simulink model "GS_model"  (R2018b)
settings: Solver=ode5  StartTime=0.0  StopTime=SimuStopTime  FixedStep=T_Simu  RelTol=1e-3
InitFcn:
  | Initial
undefined symbols (not defined in the file or in its folder): Aba10, Aba20, aeroCIP2006_S, aeroCIP2006_X, aeroCIP2006_Y, Agl0, Ass_kS, Ass_n1, Ass_n2, Ass_n3, Ass_n4, Ass_Noise, Ass_R, Ass_Resolution, Ass_TmOrder, AssA_Fix_Abs, AssB_Fix_Abs, AssC_Fix_Abs, AssD_Fix_Abs, AssE_Fix_Aps, AssF_Fix_Aps, C, c_max, c_min, Cd, CenterOfFigNX, CenterOfFigNY, CenterOfFigNZ, CenterOfFigP1, CenterOfFigP2, CenterOfFigPX, CenterOfFigPY, CenterOfFigPZ, Cmu, Crou, DEG2RAD, DiscIntNeverNeededParam, Eg_Dir, Eg_F, Eg_PrepareTime, Eg_r_L_L, Fw_Abf, Fw_Hmax, Fw_J, Fw_Spd0, Fw_Tmax, git_hash_BaseLine, git_hash_Project, Gnss_Noise_Pos, Gnss_Noise_Vel, Gnss_PropgationTime, GyroA_Fix_Abg, GyroA_Noise, GyroB_Fix_Abg, GyroB_Noise, GyroC_Fix_Abg, GyroC_Noise, GyroD_Fix_Abg, GyroD_Noise, h ... (+94)
libraries: simulink x308, sharedutil x46, aerolibutil x37, sharedtransform x31, vrlib x14, aerolibgravity2 x2
(part 19 of 20)

== matlab function GS_model/Subsystem2/Subsystem/Actuator/Motor/SADA/MATLAB Function4 ==
  settings: updateMethod=DISCRETE
  data: Tc_level output; u input; InitialAgl output
function [Tc_level , InitialAgl] =Initial(u)
Tc_AglSetEnable = u(1);
Tc_AglSetValue = u(2:7);
Tc_Reset = u(8);
Tc_Reset_Agl = u(9:14);
DataSource = u(15:20);
Agl_FC = u(21:26);
%% 输入变量、局部变量定义
persistent Tc_AglSetEnable_last DATA_Motor_Agl;

if isempty(Tc_AglSetEnable_last) || Tc_Reset == 1    %3322
    Tc_AglSetEnable_last = 0;
end
if isempty(DATA_Motor_Agl) || Tc_Reset == 1    %3322
    DATA_Motor_Agl = [0;0;0;0;0;0];
end
%% 动力学初始角度设置
if Tc_AglSetEnable_last == 0 && Tc_AglSetEnable == 1  %动力学遥控 
    Tc = [1;1;1;1;1;1];
    DATA_Motor_Agl = Tc_AglSetValue;
elseif Tc_Reset == 1 
    Tc = [1;1;1;1;1;1];
    DATA_Motor_Agl = Tc_Reset_Agl;
else
    Tc = double(DataSource==[1;1;1;1;1;1]);
    for i = 1:6
        if Tc(i) == 1 % 真采集时，取反测值
            DATA_Motor_Agl(i)  = Agl_FC(i);
        end
    end
end

Tc_AglSetEnable_last = Tc_AglSetEnable;
InitialAgl= DATA_Motor_Agl;
Tc_level =Tc;
end

== matlab function GS_model/Subsystem2/Subsystem/Actuator/Motor/QV/MATLAB Function4 ==
  settings: updateMethod=DISCRETE
  data: Tc_level output; u input; InitialAgl output
function [Tc_level , InitialAgl] =Initial(u)
Tc_AglSetEnable = u(1);
Tc_AglSetValue = u(2:5);
Tc_Reset = u(6);
Tc_Reset_Agl = u(7:10);
DataSource = u(11:14);
Agl_FC = u(15:18);
%% 输入变量、局部变量定义
persistent Tc_AglSetEnable_last DATA_Motor_Agl;

if isempty(Tc_AglSetEnable_last) || Tc_Reset == 1    %3322
    Tc_AglSetEnable_last = 0;
end
if isempty(DATA_Motor_Agl) || Tc_Reset == 1    %3322
    DATA_Motor_Agl = [0;0;0;0];
end
%% 动力学初始角度设置
if Tc_AglSetEnable_last == 0 && Tc_AglSetEnable == 1  %动力学遥控 
    Tc = [1;1;1;1];
    DATA_Motor_Agl = Tc_AglSetValue;
elseif Tc_Reset == 1 
    Tc = [1;1;1;1];
    DATA_Motor_Agl = Tc_Reset_Agl;
else
    Tc = double(DataSource==[1;1;1;1]);
    for i = 1:4
        if Tc(i) == 1 % 真采集时，取反测值
            DATA_Motor_Agl(i)  = Agl_FC(i);
        end
    end
end

Tc_AglSetEnable_last = Tc_AglSetEnable;
InitialAgl= DATA_Motor_Agl;
Tc_level =Tc;
end

== matlab function GS_model/Subsystem2/Subsystem/Sensor/GNSS/Orbit/MATLAB Function2 ==
  data: RV_i output; Orbit input
function RV_i = Orbit2RV(Orbit)
% 瞬根轨道转惯性系RV
a = Orbit(1);
e = Orbit(2);
i = Orbit(3);
OMG = Orbit(4);
omg = Orbit(5);
f = Orbit(6);
p=a*(1-e^2);
r0=p/(1+e*cos(f));
miu = 3.9860044e14;
% v0=sqrt(mu*(2/r0-1/a));
% sg=e*sin(f)/sqrt(1+e^2+2*e*cos(f));
% cg=sqrt(1-sg^2);
x0=r0*(cos(omg+f)*cos(OMG)-sin(omg+f)*cos(i)*sin(OMG));
y0=r0*(cos(omg+f)*sin(OMG)+sin(omg+f)*cos(i)*cos(OMG));
z0=r0*sin(omg+f)*sin(i);
R_i = [x0;y0;z0];
% x0=1184844.6264962;y0=-3166067.5090052;z0=6192267.2136932;
% vx0=v0*(sg*(cos(omg+f)*cos(OMG)-sin(omg+f)*cos(i)*sin(OMG))+cg*(-sin(omg+f)*cos(OMG)-cos(omg+f)*cos(i)*sin(OMG)));% x肖业伦P53
% vy0=v0*(sg*(cos(omg+f)*sin(OMG)+sin(omg+f)*cos(i)*cos(OMG))+cg*(-sin(omg+f)*sin(OMG)+cos(omg+f)*cos(i)*cos(OMG)));
% vz0=v0*(sg*sin(omg+f)*sin(i)+cg*cos(omg+f)*sin(i));
sp=[cos(omg)*cos(OMG)-sin(omg)*sin(OMG)*cos(i);cos(omg)*sin(OMG)+sin(omg)*cos(OMG)*cos(i);sin(omg)*sin(i)];
sq=[-sin(omg)*cos(OMG)-cos(omg)*sin(OMG)*cos(i);-sin(omg)*sin(OMG)+cos(omg)*cos(OMG)*cos(i);cos(omg)*sin(i)];
vx0=sqrt(miu/a/(1-e^2))*(-sin(f)*sp(1)+(e+cos(f))*sq(1));
vy0=sqrt(miu/a/(1-e^2))*(-sin(f)*sp(2)+(e+cos(f))*sq(2));
vz0=sqrt(miu/a/(1-e^2))*(-sin(f)*sp(3)+(e+cos(f))*sq(3));
V_i = [vx0;vy0;vz0];
RV_i=[R_i;V_i];

== matlab function GS_model/Subsystem2/Subsystem/Sensor/GNSS/Orbit1/MATLAB Function2 ==
  data: RV_i output; Orbit input
function RV_i = Orbit2RV(Orbit)
% 瞬根轨道转惯性系RV
a = Orbit(1);
e = Orbit(2);
i = Orbit(3);
OMG = Orbit(4);
omg = Orbit(5);
f = Orbit(6);
p=a*(1-e^2);
r0=p/(1+e*cos(f));
miu = 3.9860044e14;
% v0=sqrt(mu*(2/r0-1/a));
% sg=e*sin(f)/sqrt(1+e^2+2*e*cos(f));
% cg=sqrt(1-sg^2);
x0=r0*(cos(omg+f)*cos(OMG)-sin(omg+f)*cos(i)*sin(OMG));
y0=r0*(cos(omg+f)*sin(OMG)+sin(omg+f)*cos(i)*cos(OMG));
z0=r0*sin(omg+f)*sin(i);
R_i = [x0;y0;z0];
% x0=1184844.6264962;y0=-3166067.5090052;z0=6192267.2136932;
% vx0=v0*(sg*(cos(omg+f)*cos(OMG)-sin(omg+f)*cos(i)*sin(OMG))+cg*(-sin(omg+f)*cos(OMG)-cos(omg+f)*cos(i)*sin(OMG)));% x肖业伦P53
% vy0=v0*(sg*(cos(omg+f)*sin(OMG)+sin(omg+f)*cos(i)*cos(OMG))+cg*(-sin(omg+f)*sin(OMG)+cos(omg+f)*cos(i)*cos(OMG)));
% vz0=v0*(sg*sin(omg+f)*sin(i)+cg*cos(omg+f)*sin(i));
sp=[cos(omg)*cos(OMG)-sin(omg)*sin(OMG)*cos(i);cos(omg)*sin(OMG)+sin(omg)*cos(OMG)*cos(i);sin(omg)*sin(i)];
sq=[-sin(omg)*cos(OMG)-cos(omg)*sin(OMG)*cos(i);-sin(omg)*sin(OMG)+cos(omg)*cos(OMG)*cos(i);cos(omg)*sin(i)];
vx0=sqrt(miu/a/(1-e^2))*(-sin(f)*sp(1)+(e+cos(f))*sq(1));
vy0=sqrt(miu/a/(1-e^2))*(-sin(f)*sp(2)+(e+cos(f))*sq(2));
vz0=sqrt(miu/a/(1-e^2))*(-sin(f)*sp(3)+(e+cos(f))*sq(3));
V_i = [vx0;vy0;vz0];
RV_i=[R_i;V_i];

== matlab function GS_model/Subsystem2/Subsystem/PhysicsModel/Orbit/Subsystem1/DcmECI2ECEF ==
  data: aeroCIP2006_Y input; aeroCIP2006_X input; aeroCIP2006_S input; polarMotion input; deltaUT1 input; dCIP input; deltaAT input; Seconds input; y output
function y = fcn(aeroCIP2006_Y, aeroCIP2006_X, aeroCIP2006_S, polarMotion, deltaUT1, dCIP, deltaAT, Seconds)
UTC = add_seconds_to_date(Seconds);
UTC=UTC';
year = UTC(1,1);
month = UTC(2,1);
day = UTC(3,1);
hour = UTC(4,1);
min = UTC(5,1);
sec = UTC(6,1);

% 检查日期格式
if any(mod(year,1)~=0)
    year = fix(year);
end
if any(mod(month,1)~=0)
    month = fix(month);
end
if any(mod(day,1)~=0)
    day = fix(day);
end
if any(mod(hour,1)~=0)
    hour = fix(hour);
end
if any(mod(min,1)~=0)
    min = fix(min);
end
len = 1;

% Julian date for terrestrial time
ssUT = sec + deltaUT1; 
ssTT = sec + deltaAT + 32.184; 
secV1 = ssTT ;
secV2 = ssUT ;
    if ( month<= 2 ) % January & February
        yearV1= year- 1.0;
        monthV1 = month+ 12.0;
    else 
        yearV1=year;
        monthV1=month;
    end
dayFractionV1= (hour + min/60 + secV1/3600)/24;
dayFractionV2= (hour + min/60 + secV2/3600)/24;
dayV1 = floor( 365.25*yearV1 ) + floor( 30.6001*( monthV1 + 1.0)) + 2.0 - ...
    floor( yearV1/100.0 ) + floor( floor( yearV1/100.0 )/4.0 ) + day + ...
     - 679006.0;
% Julian date for terrestrial time
jdTT = dayFractionV1 + dayV1;
% Number of Julian centuries since J2000 for terrestrial time.
tTT = (jdTT - 51544.5)/36525;
tTT2 = tTT.*tTT;
tTT3 = tTT2.*tTT;
tTT = tTT';
tTT2 = tTT2';
tTT3 = tTT3';
tTT4 = tTT3.*tTT;
tTT5 = tTT4.*tTT;
% Julian date for UT1
jdUT1 =dayFractionV2 + dayV1 ;
% Elapsed Julian days since J2000
jdElapsed = jdUT1 - 51544.5;
% Julian day fraction
jdFraction = mod(jdElapsed,1);
        
        %% Polar motion
        % TIO locator
        sp = -0.000047*tTT/3600*pi/180;
        % Transformation matrix for polar motion
        WY=-polarMotion(1,1);WX=-polarMotion(2,1);
        W_Z = [cos(sp) sin(sp) 0;-sin(sp)  cos(sp) 0; 0  0 1];      
        W_Y = [cos(WY) 0 -sin(WY); 0 1  0;sin(WY) 0 cos(WY)];  
        W_X = [1  0  0;0 cos(WX) sin(WX);0 -sin(WX) cos(WX)];
        W=W_X*W_Y*W_Z;
        %% Earth rotation
        % Earth rotation angle
        thetaERA = mod(2*pi*(jdFraction + 0.7790572732640 + 0.00273781191135448*jdElapsed),2*pi);
        % Transformation matrix for earth rotation
        %R = angle2dcm(thetaERA,0,0);
        R_yaw = [cos(thetaERA) sin(thetaERA) 0;-sin(thetaERA)  cos(thetaERA) 0; 0  0 1];      
        R_pitch = [cos(0) 0 -sin(0); 0 1  0;sin(0) 0 cos(0)];  
        R_roll = [1  0  0;0 cos(0) sin(0);0 -sin(0) cos(0)];
        R = R_yaw * R_pitch * R_roll;
        %% Celestial Motion of the CIP
        % Arguments for lunisolar nutation
        mMoon = 485868.249036 + 1717915923.2178*tTT + 31.8792*tTT2 + 0.051635*tTT3 - 0.00024470*tTT4;
        mSun = 1287104.793048 + 129596581.0481*tTT - 0.5532*tTT2 + 0.000136*tTT3 - 0.00001149*tTT4;
        umMoon = 335779.526232 + 1739527262.8478*tTT - 12.7512*tTT2 - 0.001037*tTT3 + 0.00000417*tTT4;
        dSun = 1072260.703692 + 1602961601.2090*tTT - 6.3706*tTT2 + 0.006593*tTT3 - 0.00003169*tTT4;
        omegaMoon = 450160.398036 - 6962890.5431*tTT + 7.4722*tTT2 + 0.007702*tTT3 - 0.00005939*tTT4;
        % Arguments for planetary nutation
        lMercury = 4.402608842 + 2608.7903141574*tTT;
        lVenus = 3.176146697 + 1021.3285546211*tTT;
        lEarth = 1.753470314 + 628.3075849991*tTT;
        lMars = 6.203480913 + 334.06124267*tTT;
        lJupiter = 0.599546497 + 52.9690962641*tTT;
        lSaturn = 0.874016757 + 21.329910496*tTT;
        lUranus = 5.481293872 + 7.4781598567*tTT;
        lNeptune = 5.311886287 + 3.8133035638*tTT;
        pa = 0.02438175*tTT + 0.00000538691*tTT2;
        % Vector arrangement for series evaluation
        REconvang=[mMoon; mSun; umMoon; dSun; omegaMoon]/3600*pi/180;
        nutationV = mod([REconvang; ...
            lMercury; lVenus; lEarth; lMars; lJupiter; lSaturn; lUranus; lNeptune; pa],2*pi);
                
        % Coordinates of the CIP in the ICRS
        % Series data (according to Table 5.2a, 5.2b, and Table 5.2d)

        % Polynomial part of X and Y
        X0 = -16617 + 2004191898*tTT - 429782.9*tTT2 - 198618.34*tTT3 + 7.578*tTT4 + 5.9285*tTT5;
        Y0 = -6951 - 25896*tTT - 22407274.7*tTT2 + 1900.59*tTT3 + 1112.526*tTT4 + 0.1358*tTT5;
        % Polynomial part of S
        S0 = 94 + 3808.65*tTT - 122.68*tTT2 - 72574.11*tTT3 + 27.98*tTT4 + 15.62*tTT5;
        % Series evaluation
        % For X:
        FX = zeros(length(aeroCIP2006_X),len);
        FX(1:1306,:) = ones(1306,len);
        FX(1307:1559,:) = repmat(tTT,[253 1]);
        FX(1560:1595,:) = repmat(tTT2,[36 1]);
        FX(1596:1599,:) = repmat(tTT3,[4 1]);
        FX(1600,:) = tTT4;
        argX = aeroCIP2006_X(:,4:17)*nutationV;
        % 初始化 X 的值
        resultX = zeros(size(argX, 1), 1);  % 初始化结果向量
        for k = 1:len
            % 计算当前 k 对应的值并加到结果向量中
            resultX = resultX + (aeroCIP2006_X(:,2).*sin(argX(:,k)) + aeroCIP2006_X(:,3).*cos(argX(:,k))).*FX(:,k);
        end
        X = sum(resultX);  % 对结果向量求和得到最终结果

        FY = zeros(length(aeroCIP2006_Y),len);
        FY(1:962,:) = ones(962,len);
        FY(963:1239,:) = repmat(tTT,[277 1]);
        FY(1240:1269,:) = repmat(tTT2,[30 1]);
        FY(1270:1274,:) = repmat(tTT3,[5 1]);
        FY(1275,:) = tTT4;
        argY = aeroCIP2006_Y(:,4:17)*nutationV;
        Y = zeros(size(argY, 1), 1);  % 初始化结果向量
        for k = 1:len
            % 计算当前 k 对应的值并累加到结果向量中
            Y = Y + (aeroCIP2006_Y(:,2).*sin(argY(:,k)) + aeroCIP2006_Y(:,3).*cos(argY(:,k))).*FY(:,k);
        end
        Y = sum(Y);  % 对结果向量求和得到最终结果

        FS = zeros(length(aeroCIP2006_S),len);
        FS(1:33,:) = ones(33,len);
        FS(34:36,:) = repmat(tTT,[3 1]);
        FS(37:61,:) = repmat(tTT2,[25 1]);
        FS(62:65,:) = repmat(tTT3,[4 1]);
        FS(66,:) = tTT4;
        argS = aeroCIP2006_S(:,4:11)*[nutationV(1:5,:);nutationV(7:8,:);nutationV(14,:)];
        S = zeros(size(argS, 1), 1);  % 初始化结果向量
        for k = 1:len
            % 计算当前 k 对应的值并累加到结果向量中
            S = S + (aeroCIP2006_S(:,2).*sin(argS(:,k)) + aeroCIP2006_S(:,3).*cos(argS(:,k))).*FS(:,k);
        end
        S = sum(S);  % 对结果向量求和得到最终结果

        X = X + X0;
        Y = Y + Y0;
        S = S + S0;
        % Convert from microarcseconds to radians
        X = X*1e-6/3600*pi/180 + dCIP(1,1)';
        Y = Y*1e-6/3600*pi/180 + dCIP(2,1)';
        S = S*1e-6/3600*pi/180-X.*Y/2;
        % Coordinates of the CIP
        E = atan2(Y,X);
        d = atan(sqrt((X.^2+Y.^2)./(1-X.^2-Y.^2)));
        % Transformation matrix for celestial motion of the CIP
        %Q = angle2dcm(E,d,-E-S,'ZYZ');
        Q_yaw = [cos(-E-S) sin(-E-S) 0;-sin(-E-S)  cos(-E-S) 0; 0  0 1];
        Q_pitch = [cos(d) 0 -sin(d); 0 1  0;sin(d) 0 cos(d)];
        Q_roll = [cos(E) sin(E) 0;-sin(E)  cos(E) 0; 0  0 1];
        Q = Q_yaw * Q_pitch * Q_roll;
        %% Matrix calculations
        tmp = cell(1, len);
        
        % 进行循环计算
        for k = 1:len
            tmp{k} = W(:,:,k) * R(:,:,k) * Q(:,:,k);
        end
        %DCM = reshape(cell2mat(tmp),3,3,len);
        % 初始化 DCM 矩阵
        DCM = zeros(3, 3, len);      
        % 循环计算每个 tmp 单元格并填充到 DCM 矩阵中
        for k = 1:len
            % 计算旋转矩阵并填充到 DCM 中
            DCM(:,:,k) = W(:,:,k) * R(:,:,k) * Q(:,:,k);
        end
function new_date = add_seconds_to_date(seconds)
    % 初始日期
    initial_date = [1970, 1, 1, 0, 0, 0]; % [年, 月, 日, 时, 分, 秒]

    % 计算新日期
    new_date = initial_date;

    % 添加秒数
    new_date(6) = new_date(6) + seconds; % 秒数相加

    % 处理秒数超过60的情况
    if new_date(6) >= 60
        new_date(5) = new_date(5) + floor(new_date(6) / 60); % 分钟数相加
        new_date(6) = mod(new_date(6), 60); % 更新秒数
    end

    % 处理分钟数超过60的情况
    if new_date(5) >= 60
        new_date(4) = new_date(4) + floor(new_date(5) / 60); % 小时数相加
        new_date(5) = mod(new_date(5), 60); % 更新分钟数
    end

    % 处理小时数超过24的情况
    if new_date(4) >= 24
        new_date(3) = new_date(3) + floor(new_date(4) / 24); % 天数相加
        new_date(4) = mod(new_date(4), 24); % 更新小时数
    end

    % 处理月份和年份的变化
    while new_date(3) > days_in_month(new_date(1), new_date(2)) % 天数大于该月的天数
        new_date(3) = new_date(3) - days_in_month(new_date(1), new_date(2)); % 减去该月的天数
        new_date(2) = new_date(2) + 1; % 月份加一

        % 处理月份超过12的情况
        if new_date(2) > 12
            new_date(1) = new_date(1) + 1; % 年份加一
            new_date(2) = 1; % 月份重置为1
        end
    end


    % 嵌套函数：根据年份和月份计算该月的天数
    function days = days_in_month(year, month)
        if month == 2
            if is_leap_year(year)
                days = 29;
            else
                days = 28;
            end
        elseif ismember(month, [4, 6, 9, 11])
            days = 30;
        else
            days = 31;
        end
    end

    % 嵌套函数：判断是否为闰年
    function leap = is_leap_year(year)
        leap = mod(year, 4) == 0 && (mod(year, 100) ~= 0 || mod(year, 400) == 0);
    end
end
function normalized_angle = normalize_angle1(angle)
    normalized_angle = mod(angle, 2*pi);
    normalized_angle(normalized_angle == 0) = 2*pi;
end
function normalized_angles = normalize_angle2(angles)
    % 将数组中的每个弧度角转换到 (0, 2π) 范围内
    % 输入:
    %   angles - 任意弧度角数组，可以是标量、向量或矩阵
    % 输出:
    %   normalized_angles - 在 (0, 2π) 范围内的等效弧度角数组
    
    % 使用mod函数将角度转换到 [0, 2π) 范围内
    normalized_angles = mod(angles, 2*pi);
    
    % 将范围 [0, 2π) 变为 (0, 2π)，如果需要的话
    normalized_angles(normalized_angles == 0) = 2*pi;
end

y = DCM;
end

== matlab function GS_model/Subsystem2/Subsystem/Sensor/GNSS/Orbit/Subsystem1/MATLAB Function ==
  data: Utc input; A_GI output
function A_GI = Matrix_J2000toG84(Utc)
Tjc = (((Utc-1609459200)/86400+2459215.5)-2451545.0)/36525;
zetaA=(2306.2181*Tjc+0.30188*Tjc^2)/3600/180*pi;
zA=(2306.2181*Tjc+1.09468*Tjc^2)/3600/180*pi;
thetaA=(2004.3109*Tjc-0.42665*Tjc^2)/3600/180*pi;
RP=angle2dcm(-zetaA,thetaA,-zA,'ZYZ');
Omg_M=mod(125.044555556-1934.1361850*Tjc,360)/180*pi;
eps=0.409036061380284;
deltaRA=-17.2*sin(Omg_M)/3600/180*pi;
deltaeps=9.202*cos(Omg_M)/3600/180*pi;
RN=[cos(deltaRA*sin(eps)) 0 -sin(deltaRA*sin(eps));...
    -sin(deltaeps)*sin(deltaRA*sin(eps)) cos(deltaeps) -sin(deltaeps)*cos(deltaRA*sin(eps));...
    cos(deltaeps)*sin(deltaRA*sin(eps)) sin(deltaeps) cos(deltaeps)*cos(deltaRA*sin(eps))];
Theta=(mod(280.46061837+360.98564736629*Tjc*36525,360))/180*pi;
RS=[cos(Theta) sin(Theta) 0;-sin(Theta) cos(Theta) 0;0 0 1];
RM=eye(3);
A_GI = RM*RS*RN*RP;

function dcm = angle2dcm( r1, r2, r3, varargin )
%  ANGLE2DCM Create direction cosine matrix from rotation angles.
%   N = ANGLE2DCM( R1, R2, R3 ) calculates the direction cosine matrix, N,
%   for a given set of rotation angles, R1, R2, R3.   R1 is an M array of
%   first rotation angles.  R2 is an M array of second rotation angles.  R3
%   is an M array of third rotation angles.  N returns an 3-by-3-by-M
%   matrix containing M direction cosine matrices.  Rotation angles are
%   input in radians.  
%
%   N = ANGLE2DCM( R1, R2, R3, S ) calculates the direction cosine matrix,
%   N, for a given set of rotation angles, R1, R2, R3, and a specified
%   rotation sequence, S. 
%
%   The default rotation sequence is 'ZYX' where the order of rotation
%   angles for the default rotation are R1 = Z Axis Rotation, R2 = Y Axis
%   Rotation, and R3 = X Axis Rotation. 
%
%   All rotation sequences, S, are supported: 'ZYX', 'ZYZ', 'ZXY', 'ZXZ',
%   'YXZ', 'YXY', 'YZX', 'YZY', 'XYZ', 'XYX', 'XZY', and 'XZX'.
%
%   Examples:
%
%   Determine the direction cosine matrix from rotation angles:
%      yaw = 0.7854; 
%      pitch = 0.1; 
%      roll = 0;
%      dcm = angle2dcm( yaw, pitch, roll )
%
%   Determine the direction cosine matrix from multiple rotation angles:
%      yaw = [0.7854 0.5]; 
%      pitch = [0.1 0.3]; 
%      roll = [0 0.1];
%      dcm = angle2dcm( pitch, roll, yaw, 'YXZ' )
%
%   See also DCM2ANGLE, DCM2QUAT, QUAT2DCM, QUAT2ANGLE.

%   Copyright 2000-2016 The MathWorks, Inc.

narginchk(3,4)

if any(~isreal(r1) || ~isnumeric(r1))
    error(message('aero:angle2dcm:isNotReal1'));
end

if any(~isreal(r2) || ~isnumeric(r2))
    error(message('aero:angle2dcm:isNotReal2'));
end

if any(~isreal(r3) || ~isnumeric(r3))
    error(message('aero:angle2dcm:isNotReal3'));
end

if (length(r1) ~= length(r2)) || (length(r1) ~= length(r3))
    error(message('aero:angle2dcm:wrongDimension'));
end

if nargin == 3
    type = 'zyx';
else
    if ischar( varargin{1} ) || isstring(varargin{1})
        type = char(varargin{1});
    else
        error(message('aero:angle2dcm:notChar'));
    end
end

angles = [r1(:) r2(:) r3(:)];

dcm = zeros(3,3,size(angles,1));
cang = cos( angles );
sang = sin( angles );

switch lower( type )
    case 'zyx'
        %     [          cy*cz,          cy*sz,            -sy]
        %     [ sy*sx*cz-sz*cx, sy*sx*sz+cz*cx,          cy*sx]
        %     [ sy*cx*cz+sz*sx, sy*cx*sz-cz*sx,          cy*cx]

        dcm(1,1,:) = cang(:,2).*cang(:,1);
        dcm(1,2,:) = cang(:,2).*sang(:,1);
        dcm(1,3,:) = -sang(:,2);
        dcm(2,1,:) = sang(:,3).*sang(:,2).*cang(:,1) - cang(:,3).*sang(:,1);
        dcm(2,2,:) = sang(:,3).*sang(:,2).*sang(:,1) + cang(:,3).*cang(:,1);
        dcm(2,3,:) = sang(:,3).*cang(:,2);
        dcm(3,1,:) = cang(:,3).*sang(:,2).*cang(:,1) + sang(:,3).*sang(:,1);
        dcm(3,2,:) = cang(:,3).*sang(:,2).*sang(:,1) - sang(:,3).*cang(:,1);
        dcm(3,3,:) = cang(:,3).*cang(:,2);

    case 'zyz'
        %     [  cz2*cy*cz-sz2*sz,  cz2*cy*sz+sz2*cz,           -cz2*sy]
        %     [ -sz2*cy*cz-cz2*sz, -sz2*cy*sz+cz2*cz,            sz2*sy]
        %     [             sy*cz,             sy*sz,                cy]
        
        dcm(1,1,:) = cang(:,1).*cang(:,3).*cang(:,2) - sang(:,1).*sang(:,3);
        dcm(1,2,:) = sang(:,1).*cang(:,3).*cang(:,2) + cang(:,1).*sang(:,3);
        dcm(1,3,:) = -sang(:,2).*cang(:,3);  
        dcm(2,1,:) = -cang(:,1).*cang(:,2).*sang(:,3) - sang(:,1).*cang(:,3);                
        dcm(2,2,:) = -sang(:,1).*cang(:,2).*sang(:,3) + cang(:,1).*cang(:,3);
        dcm(2,3,:) = sang(:,2).*sang(:,3);     
        dcm(3,1,:) = cang(:,1).*sang(:,2);
        dcm(3,2,:) = sang(:,1).*sang(:,2);  
        dcm(3,3,:) = cang(:,2);
                
    case 'zxy'
        %     [ cy*cz-sy*sx*sz, cy*sz+sy*sx*cz,         -sy*cx]
        %     [         -sz*cx,          cz*cx,             sx]
        %     [ sy*cz+cy*sx*sz, sy*sz-cy*sx*cz,          cy*cx]

        dcm(1,1,:) = cang(:,3).*cang(:,1) - sang(:,2).*sang(:,3).*sang(:,1);
        dcm(1,2,:) = cang(:,3).*sang(:,1) + sang(:,2).*sang(:,3).*cang(:,1);
        dcm(1,3,:) = -sang(:,3).*cang(:,2);
        dcm(2,1,:) = -cang(:,2).*sang(:,1);
        dcm(2,2,:) = cang(:,2).*cang(:,1);
        dcm(2,3,:) = sang(:,2);
        dcm(3,1,:) = sang(:,3).*cang(:,1) + sang(:,2).*cang(:,3).*sang(:,1);
        dcm(3,2,:) = sang(:,3).*sang(:,1) - sang(:,2).*cang(:,3).*cang(:,1);
        dcm(3,3,:) = cang(:,2).*cang(:,3);

    case 'zxz'
        %     [  cz2*cz-sz2*cx*sz,  cz2*sz+sz2*cx*cz,            sz2*sx]
        %     [ -sz2*cz-cz2*cx*sz, -sz2*sz+cz2*cx*cz,            cz2*sx]
        %     [             sz*sx,            -cz*sx,                cx]

        dcm(1,1,:) = -sang(:,1).*cang(:,2).*sang(:,3) + cang(:,1).*cang(:,3);
        dcm(1,2,:) = cang(:,1).*cang(:,2).*sang(:,3) + sang(:,1).*cang(:,3);                
        dcm(1,3,:) = sang(:,2).*sang(:,3);     
        dcm(2,1,:) = -sang(:,1).*cang(:,3).*cang(:,2) - cang(:,1).*sang(:,3);
        dcm(2,2,:) = cang(:,1).*cang(:,3).*cang(:,2) - sang(:,1).*sang(:,3);
        dcm(2,3,:) = sang(:,2).*cang(:,3);  
        dcm(3,1,:) = sang(:,1).*sang(:,2);  
        dcm(3,2,:) = -cang(:,1).*sang(:,2);
        dcm(3,3,:) = cang(:,2);

    case 'yxz'
        %     [  cy*cz+sy*sx*sz,           sz*cx, -sy*cz+cy*sx*sz]
        %     [ -cy*sz+sy*sx*cz,           cz*cx,  sy*sz+cy*sx*cz]
        %     [           sy*cx,             -sx,           cy*cx]

        dcm(1,1,:) = cang(:,1).*cang(:,3) + sang(:,2).*sang(:,1).*sang(:,3);
        dcm(1,2,:) = cang(:,2).*sang(:,3);
        dcm(1,3,:) = -sang(:,1).*cang(:,3) + sang(:,2).*cang(:,1).*sang(:,3);
        dcm(2,1,:) = -cang(:,1).*sang(:,3) + sang(:,2).*sang(:,1).*cang(:,3);
        dcm(2,2,:) = cang(:,2).*cang(:,3);
        dcm(2,3,:) = sang(:,1).*sang(:,3) + sang(:,2).*cang(:,1).*cang(:,3);        
        dcm(3,1,:) = sang(:,1).*cang(:,2);
        dcm(3,2,:) = -sang(:,2);
        dcm(3,3,:) = cang(:,2).*cang(:,1);

    case 'yxy'
        %     [  cy2*cy-sy2*cx*sy,            sy2*sx, -cy2*sy-sy2*cx*cy]
        %     [             sy*sx,                cx,             cy*sx]
        %     [  sy2*cy+cy2*cx*sy,           -cy2*sx, -sy2*sy+cy2*cx*cy]

        dcm(1,1,:) = -sang(:,1).*cang(:,2).*sang(:,3) + cang(:,1).*cang(:,3);
        dcm(1,2,:) = sang(:,2).*sang(:,3);     
        dcm(1,3,:) = -cang(:,1).*cang(:,2).*sang(:,3) - sang(:,1).*cang(:,3);                
        dcm(2,1,:) = sang(:,1).*sang(:,2);  
        dcm(2,2,:) = cang(:,2);
        dcm(2,3,:) = cang(:,1).*sang(:,2);
        dcm(3,1,:) = sang(:,1).*cang(:,3).*cang(:,2) + cang(:,1).*sang(:,3);
        dcm(3,2,:) = -sang(:,2).*cang(:,3);  
        dcm(3,3,:) = cang(:,1).*cang(:,3).*cang(:,2) - sang(:,1).*sang(:,3);
        
    case 'yzx'
        %     [           cy*cz,              sz,          -sy*cz]
        %     [ -sz*cx*cy+sy*sx,           cz*cx,  sy*cx*sz+cy*sx]
        %     [  cy*sx*sz+sy*cx,          -cz*sx, -sy*sx*sz+cy*cx]

        dcm(1,1,:) = cang(:,1).*cang(:,2);
        dcm(1,2,:) = sang(:,2);
        dcm(1,3,:) = -sang(:,1).*cang(:,2);
        dcm(2,1,:) = -cang(:,3).*cang(:,1).*sang(:,2) + sang(:,3).*sang(:,1);
        dcm(2,2,:) = cang(:,2).*cang(:,3);
        dcm(2,3,:) = cang(:,3).*sang(:,1).*sang(:,2) + sang(:,3).*cang(:,1);        
        dcm(3,1,:) = sang(:,3).*cang(:,1).*sang(:,2) + cang(:,3).*sang(:,1);
        dcm(3,2,:) = -sang(:,3).*cang(:,2);
        dcm(3,3,:) = -sang(:,3).*sang(:,1).*sang(:,2) + cang(:,3).*cang(:,1);
        
    case 'yzy'
        %     [  cy2*cz*cy-sy2*sy,            cy2*sz, -cy2*cz*sy-sy2*cy]
        %     [            -cy*sz,                cz,             sy*sz]
        %     [  sy2*cz*cy+cy2*sy,            sy2*sz, -sy2*cz*sy+cy2*cy]

        dcm(1,1,:) = cang(:,1).*cang(:,3).*cang(:,2) - sang(:,1).*sang(:,3);
        dcm(1,2,:) = sang(:,2).*cang(:,3);  
        dcm(1,3,:) = -sang(:,1).*cang(:,3).*cang(:,2) - cang(:,1).*sang(:,3);
        dcm(2,1,:) = -cang(:,1).*sang(:,2);
        dcm(2,2,:) = cang(:,2);
        dcm(2,3,:) = sang(:,1).*sang(:,2);  
        dcm(3,1,:) = cang(:,1).*cang(:,2).*sang(:,3) + sang(:,1).*cang(:,3);                
        dcm(3,2,:) = sang(:,2).*sang(:,3);     
        dcm(3,3,:) = -sang(:,1).*cang(:,2).*sang(:,3) + cang(:,1).*cang(:,3);

    case 'xyz'
        %     [          cy*cz, sz*cx+sy*sx*cz, sz*sx-sy*cx*cz]
        %     [         -cy*sz, cz*cx-sy*sx*sz, cz*sx+sy*cx*sz]
        %     [             sy,         -cy*sx,          cy*cx]

        dcm(1,1,:) = cang(:,2).*cang(:,3);
        dcm(1,2,:) = sang(:,1).*sang(:,2).*cang(:,3) + cang(:,1).*sang(:,3);
        dcm(1,3,:) = -cang(:,1).*sang(:,2).*cang(:,3) + sang(:,1).*sang(:,3);
        dcm(2,1,:) = -cang(:,2).*sang(:,3);
        dcm(2,2,:) = -sang(:,1).*sang(:,2).*sang(:,3) + cang(:,1).*cang(:,3);
        dcm(2,3,:) = cang(:,1).*sang(:,2).*sang(:,3) + sang(:,1).*cang(:,3);        
        dcm(3,1,:) = sang(:,2);
        dcm(3,2,:) = -sang(:,1).*cang(:,2);
        dcm(3,3,:) = cang(:,1).*cang(:,2);
        
    case 'xyx'
        %     [                cy,             sy*sx,            -sy*cx]
        %     [            sx2*sy,  cx2*cx-sx2*cy*sx,  cx2*sx+sx2*cy*cx]
        %     [            cx2*sy, -sx2*cx-cx2*cy*sx, -sx2*sx+cx2*cy*cx]

        dcm(1,1,:) = cang(:,2);
        dcm(1,2,:) = sang(:,1).*sang(:,2);     
        dcm(1,3,:) = -cang(:,1).*sang(:,2);
        dcm(2,1,:) = sang(:,2).*sang(:,3);        
        dcm(2,2,:) = -sang(:,1).*cang(:,2).*sang(:,3) + cang(:,1).*cang(:,3);
        dcm(2,3,:) = cang(:,1).*cang(:,2).*sang(:,3) + sang(:,1).*cang(:,3);                
        dcm(3,1,:) = sang(:,2).*cang(:,3);        
        dcm(3,2,:) = -sang(:,1).*cang(:,3).*cang(:,2) - cang(:,1).*sang(:,3);
        dcm(3,3,:) = cang(:,1).*cang(:,3).*cang(:,2) - sang(:,1).*sang(:,3);
        
    case 'xzy'
        %     [          cy*cz, sz*cx*cy+sy*sx, cy*sx*sz-sy*cx]
        %     [            -sz,          cz*cx,          cz*sx]
        %     [          sy*cz, sy*cx*sz-cy*sx, sy*sx*sz+cy*cx]

        dcm(1,1,:) = cang(:,3).*cang(:,2);
        dcm(1,2,:) = cang(:,1).*cang(:,3).*sang(:,2) + sang(:,1).*sang(:,3);
        dcm(1,3,:) = sang(:,1).*cang(:,3).*sang(:,2) - cang(:,1).*sang(:,3);
        dcm(2,1,:) = -sang(:,2);
        dcm(2,2,:) = cang(:,1).*cang(:,2);
        dcm(2,3,:) = sang(:,1).*cang(:,2);        
        dcm(3,1,:) = sang(:,3).*cang(:,2);
        dcm(3,2,:) = cang(:,1).*sang(:,2).*sang(:,3) - sang(:,1).*cang(:,3);                
        dcm(3,3,:) = sang(:,1).*sang(:,2).*sang(:,3) + cang(:,1).*cang(:,3);
        
    case 'xzx'
        %     [                cz,             sz*cx,             sz*sx]
        %     [           -cx2*sz,  cx2*cz*cx-sx2*sx,  cx2*cz*sx+sx2*cx]
        %     [            sx2*sz, -sx2*cz*cx-cx2*sx, -sx2*cz*sx+cx2*cx]

        dcm(1,1,:) = cang(:,2);
        dcm(1,2,:) = cang(:,1).*sang(:,2);     
        dcm(1,3,:) = sang(:,1).*sang(:,2);
        dcm(2,1,:) = -sang(:,2).*cang(:,3);        
        dcm(2,2,:) = cang(:,1).*cang(:,3).*cang(:,2) - sang(:,1).*sang(:,3);
        dcm(2,3,:) = sang(:,1).*cang(:,3).*cang(:,2) + cang(:,1).*sang(:,3);
        dcm(3,1,:) = sang(:,2).*sang(:,3);
        dcm(3,2,:) = -cang(:,1).*cang(:,2).*sang(:,3) - sang(:,1).*cang(:,3);                
        dcm(3,3,:) = -sang(:,1).*cang(:,2).*sang(:,3) + cang(:,1).*cang(:,3);

    otherwise
        error(message('aero:angle2dcm:unknownRotation', type));
end

== matlab function GS_model/Subsystem2/Subsystem/Sensor/GNSS/Orbit1/Subsystem1/MATLAB Function ==
  data: Utc input; A_GI output
function A_GI = Matrix_J2000toG84(Utc)
Tjc = (((Utc-1609459200)/86400+2459215.5)-2451545.0)/36525;
zetaA=(2306.2181*Tjc+0.30188*Tjc^2)/3600/180*pi;
zA=(2306.2181*Tjc+1.09468*Tjc^2)/3600/180*pi;
thetaA=(2004.3109*Tjc-0.42665*Tjc^2)/3600/180*pi;
RP=angle2dcm(-zetaA,thetaA,-zA,'ZYZ');
Omg_M=mod(125.044555556-1934.1361850*Tjc,360)/180*pi;
eps=0.409036061380284;
deltaRA=-17.2*sin(Omg_M)/3600/180*pi;
deltaeps=9.202*cos(Omg_M)/3600/180*pi;
RN=[cos(deltaRA*sin(eps)) 0 -sin(deltaRA*sin(eps));...
    -sin(deltaeps)*sin(deltaRA*sin(eps)) cos(deltaeps) -sin(deltaeps)*cos(deltaRA*sin(eps));...
    cos(deltaeps)*sin(deltaRA*sin(eps)) sin(deltaeps) cos(deltaeps)*cos(deltaRA*sin(eps))];
Theta=(mod(280.46061837+360.98564736629*Tjc*36525,360))/180*pi;
RS=[cos(Theta) sin(Theta) 0;-sin(Theta) cos(Theta) 0;0 0 1];
RM=eye(3);
A_GI = RM*RS*RN*RP;

function dcm = angle2dcm( r1, r2, r3, varargin )
%  ANGLE2DCM Create direction cosine matrix from rotation angles.
%   N = ANGLE2DCM( R1, R2, R3 ) calculates the direction cosine matrix, N,
%   for a given set of rotation angles, R1, R2, R3.   R1 is an M array of
%   first rotation angles.  R2 is an M array of second rotation angles.  R3
%   is an M array of third rotation angles.  N returns an 3-by-3-by-M
%   matrix containing M direction cosine matrices.  Rotation angles are
%   input in radians.  
%
%   N = ANGLE2DCM( R1, R2, R3, S ) calculates the direction cosine matrix,
%   N, for a given set of rotation angles, R1, R2, R3, and a specified
%   rotation sequence, S. 
%
%   The default rotation sequence is 'ZYX' where the order of rotation
%   angles for the default rotation are R1 = Z Axis Rotation, R2 = Y Axis
%   Rotation, and R3 = X Axis Rotation. 
%
%   All rotation sequences, S, are supported: 'ZYX', 'ZYZ', 'ZXY', 'ZXZ',
%   'YXZ', 'YXY', 'YZX', 'YZY', 'XYZ', 'XYX', 'XZY', and 'XZX'.
%
%   Examples:
%
%   Determine the direction cosine matrix from rotation angles:
%      yaw = 0.7854; 
%      pitch = 0.1; 
%      roll = 0;
%      dcm = angle2dcm( yaw, pitch, roll )
%
%   Determine the direction cosine matrix from multiple rotation angles:
%      yaw = [0.7854 0.5]; 
%      pitch = [0.1 0.3]; 
%      roll = [0 0.1];
%      dcm = angle2dcm( pitch, roll, yaw, 'YXZ' )
%
%   See also DCM2ANGLE, DCM2QUAT, QUAT2DCM, QUAT2ANGLE.

%   Copyright 2000-2016 The MathWorks, Inc.

narginchk(3,4)

if any(~isreal(r1) || ~isnumeric(r1))
    error(message('aero:angle2dcm:isNotReal1'));
end

if any(~isreal(r2) || ~isnumeric(r2))
    error(message('aero:angle2dcm:isNotReal2'));
end

if any(~isreal(r3) || ~isnumeric(r3))
    error(message('aero:angle2dcm:isNotReal3'));
end

if (length(r1) ~= length(r2)) || (length(r1) ~= length(r3))
    error(message('aero:angle2dcm:wrongDimension'));
end

if nargin == 3
    type = 'zyx';
else
    if ischar( varargin{1} ) || isstring(varargin{1})
        type = char(varargin{1});
    else
        error(message('aero:angle2dcm:notChar'));
    end
end

angles = [r1(:) r2(:) r3(:)];

dcm = zeros(3,3,size(angles,1));
cang = cos( angles );
sang = sin( angles );

switch lower( type )
    case 'zyx'
        %     [          cy*cz,          cy*sz,            -sy]
        %     [ sy*sx*cz-sz*cx, sy*sx*sz+cz*cx,          cy*sx]
        %     [ sy*cx*cz+sz*sx, sy*cx*sz-cz*sx,          cy*cx]

        dcm(1,1,:) = cang(:,2).*cang(:,1);
        dcm(1,2,:) = cang(:,2).*sang(:,1);
        dcm(1,3,:) = -sang(:,2);
        dcm(2,1,:) = sang(:,3).*sang(:,2).*cang(:,1) - cang(:,3).*sang(:,1);
        dcm(2,2,:) = sang(:,3).*sang(:,2).*sang(:,1) + cang(:,3).*cang(:,1);
        dcm(2,3,:) = sang(:,3).*cang(:,2);
        dcm(3,1,:) = cang(:,3).*sang(:,2).*cang(:,1) + sang(:,3).*sang(:,1);
        dcm(3,2,:) = cang(:,3).*sang(:,2).*sang(:,1) - sang(:,3).*cang(:,1);
        dcm(3,3,:) = cang(:,3).*cang(:,2);

    case 'zyz'
        %     [  cz2*cy*cz-sz2*sz,  cz2*cy*sz+sz2*cz,           -cz2*sy]
        %     [ -sz2*cy*cz-cz2*sz, -sz2*cy*sz+cz2*cz,            sz2*sy]
        %     [             sy*cz,             sy*sz,                cy]
        
        dcm(1,1,:) = cang(:,1).*cang(:,3).*cang(:,2) - sang(:,1).*sang(:,3);
        dcm(1,2,:) = sang(:,1).*cang(:,3).*cang(:,2) + cang(:,1).*sang(:,3);
        dcm(1,3,:) = -sang(:,2).*cang(:,3);  
        dcm(2,1,:) = -cang(:,1).*cang(:,2).*sang(:,3) - sang(:,1).*cang(:,3);                
        dcm(2,2,:) = -sang(:,1).*cang(:,2).*sang(:,3) + cang(:,1).*cang(:,3);
        dcm(2,3,:) = sang(:,2).*sang(:,3);     
        dcm(3,1,:) = cang(:,1).*sang(:,2);
        dcm(3,2,:) = sang(:,1).*sang(:,2);  
        dcm(3,3,:) = cang(:,2);
                
    case 'zxy'
        %     [ cy*cz-sy*sx*sz, cy*sz+sy*sx*cz,         -sy*cx]
        %     [         -sz*cx,          cz*cx,             sx]
        %     [ sy*cz+cy*sx*sz, sy*sz-cy*sx*cz,          cy*cx]

        dcm(1,1,:) = cang(:,3).*cang(:,1) - sang(:,2).*sang(:,3).*sang(:,1);
        dcm(1,2,:) = cang(:,3).*sang(:,1) + sang(:,2).*sang(:,3).*cang(:,1);
        dcm(1,3,:) = -sang(:,3).*cang(:,2);
        dcm(2,1,:) = -cang(:,2).*sang(:,1);
        dcm(2,2,:) = cang(:,2).*cang(:,1);
        dcm(2,3,:) = sang(:,2);
        dcm(3,1,:) = sang(:,3).*cang(:,1) + sang(:,2).*cang(:,3).*sang(:,1);
        dcm(3,2,:) = sang(:,3).*sang(:,1) - sang(:,2).*cang(:,3).*cang(:,1);
        dcm(3,3,:) = cang(:,2).*cang(:,3);

    case 'zxz'
        %     [  cz2*cz-sz2*cx*sz,  cz2*sz+sz2*cx*cz,            sz2*sx]
        %     [ -sz2*cz-cz2*cx*sz, -sz2*sz+cz2*cx*cz,            cz2*sx]
        %     [             sz*sx,            -cz*sx,                cx]

        dcm(1,1,:) = -sang(:,1).*cang(:,2).*sang(:,3) + cang(:,1).*cang(:,3);
        dcm(1,2,:) = cang(:,1).*cang(:,2).*sang(:,3) + sang(:,1).*cang(:,3);                
        dcm(1,3,:) = sang(:,2).*sang(:,3);     
        dcm(2,1,:) = -sang(:,1).*cang(:,3).*cang(:,2) - cang(:,1).*sang(:,3);
        dcm(2,2,:) = cang(:,1).*cang(:,3).*cang(:,2) - sang(:,1).*sang(:,3);
        dcm(2,3,:) = sang(:,2).*cang(:,3);  
        dcm(3,1,:) = sang(:,1).*sang(:,2);  
        dcm(3,2,:) = -cang(:,1).*sang(:,2);
        dcm(3,3,:) = cang(:,2);

    case 'yxz'
        %     [  cy*cz+sy*sx*sz,           sz*cx, -sy*cz+cy*sx*sz]
        %     [ -cy*sz+sy*sx*cz,           cz*cx,  sy*sz+cy*sx*cz]
        %     [           sy*cx,             -sx,           cy*cx]

        dcm(1,1,:) = cang(:,1).*cang(:,3) + sang(:,2).*sang(:,1).*sang(:,3);
        dcm(1,2,:) = cang(:,2).*sang(:,3);
        dcm(1,3,:) = -sang(:,1).*cang(:,3) + sang(:,2).*cang(:,1).*sang(:,3);
        dcm(2,1,:) = -cang(:,1).*sang(:,3) + sang(:,2).*sang(:,1).*cang(:,3);
        dcm(2,2,:) = cang(:,2).*cang(:,3);
        dcm(2,3,:) = sang(:,1).*sang(:,3) + sang(:,2).*cang(:,1).*cang(:,3);        
        dcm(3,1,:) = sang(:,1).*cang(:,2);
        dcm(3,2,:) = -sang(:,2);
        dcm(3,3,:) = cang(:,2).*cang(:,1);

    case 'yxy'
        %     [  cy2*cy-sy2*cx*sy,            sy2*sx, -cy2*sy-sy2*cx*cy]
        %     [             sy*sx,                cx,             cy*sx]
        %     [  sy2*cy+cy2*cx*sy,           -cy2*sx, -sy2*sy+cy2*cx*cy]

        dcm(1,1,:) = -sang(:,1).*cang(:,2).*sang(:,3) + cang(:,1).*cang(:,3);
        dcm(1,2,:) = sang(:,2).*sang(:,3);     
        dcm(1,3,:) = -cang(:,1).*cang(:,2).*sang(:,3) - sang(:,1).*cang(:,3);                
        dcm(2,1,:) = sang(:,1).*sang(:,2);  
        dcm(2,2,:) = cang(:,2);
        dcm(2,3,:) = cang(:,1).*sang(:,2);
        dcm(3,1,:) = sang(:,1).*cang(:,3).*cang(:,2) + cang(:,1).*sang(:,3);
        dcm(3,2,:) = -sang(:,2).*cang(:,3);  
        dcm(3,3,:) = cang(:,1).*cang(:,3).*cang(:,2) - sang(:,1).*sang(:,3);
        
    case 'yzx'
        %     [           cy*cz,              sz,          -sy*cz]
        %     [ -sz*cx*cy+sy*sx,           cz*cx,  sy*cx*sz+cy*sx]
        %     [  cy*sx*sz+sy*cx,          -cz*sx, -sy*sx*sz+cy*cx]

        dcm(1,1,:) = cang(:,1).*cang(:,2);
        dcm(1,2,:) = sang(:,2);
        dcm(1,3,:) = -sang(:,1).*cang(:,2);
        dcm(2,1,:) = -cang(:,3).*cang(:,1).*sang(:,2) + sang(:,3).*sang(:,1);
        dcm(2,2,:) = cang(:,2).*cang(:,3);
        dcm(2,3,:) = cang(:,3).*sang(:,1).*sang(:,2) + sang(:,3).*cang(:,1);        
        dcm(3,1,:) = sang(:,3).*cang(:,1).*sang(:,2) + cang(:,3).*sang(:,1);
        dcm(3,2,:) = -sang(:,3).*cang(:,2);
        dcm(3,3,:) = -sang(:,3).*sang(:,1).*sang(:,2) + cang(:,3).*cang(:,1);
        
    case 'yzy'
        %     [  cy2*cz*cy-sy2*sy,            cy2*sz, -cy2*cz*sy-sy2*cy]
        %     [            -cy*sz,                cz,             sy*sz]
        %     [  sy2*cz*cy+cy2*sy,            sy2*sz, -sy2*cz*sy+cy2*cy]

        dcm(1,1,:) = cang(:,1).*cang(:,3).*cang(:,2) - sang(:,1).*sang(:,3);
        dcm(1,2,:) = sang(:,2).*cang(:,3);  
        dcm(1,3,:) = -sang(:,1).*cang(:,3).*cang(:,2) - cang(:,1).*sang(:,3);
        dcm(2,1,:) = -cang(:,1).*sang(:,2);
        dcm(2,2,:) = cang(:,2);
        dcm(2,3,:) = sang(:,1).*sang(:,2);  
        dcm(3,1,:) = cang(:,1).*cang(:,2).*sang(:,3) + sang(:,1).*cang(:,3);                
        dcm(3,2,:) = sang(:,2).*sang(:,3);     
        dcm(3,3,:) = -sang(:,1).*cang(:,2).*sang(:,3) + cang(:,1).*cang(:,3);

    case 'xyz'
        %     [          cy*cz, sz*cx+sy*sx*cz, sz*sx-sy*cx*cz]
        %     [         -cy*sz, cz*cx-sy*sx*sz, cz*sx+sy*cx*sz]
        %     [             sy,         -cy*sx,          cy*cx]

        dcm(1,1,:) = cang(:,2).*cang(:,3);
        dcm(1,2,:) = sang(:,1).*sang(:,2).*cang(:,3) + cang(:,1).*sang(:,3);
        dcm(1,3,:) = -cang(:,1).*sang(:,2).*cang(:,3) + sang(:,1).*sang(:,3);
        dcm(2,1,:) = -cang(:,2).*sang(:,3);
        dcm(2,2,:) = -sang(:,1).*sang(:,2).*sang(:,3) + cang(:,1).*cang(:,3);
        dcm(2,3,:) = cang(:,1).*sang(:,2).*sang(:,3) + sang(:,1).*cang(:,3);        
        dcm(3,1,:) = sang(:,2);
        dcm(3,2,:) = -sang(:,1).*cang(:,2);
        dcm(3,3,:) = cang(:,1).*cang(:,2);
        
    case 'xyx'
        %     [                cy,             sy*sx,            -sy*cx]
        %     [            sx2*sy,  cx2*cx-sx2*cy*sx,  cx2*sx+sx2*cy*cx]
        %     [            cx2*sy, -sx2*cx-cx2*cy*sx, -sx2*sx+cx2*cy*cx]

        dcm(1,1,:) = cang(:,2);
        dcm(1,2,:) = sang(:,1).*sang(:,2);     
        dcm(1,3,:) = -cang(:,1).*sang(:,2);
        dcm(2,1,:) = sang(:,2).*sang(:,3);        
        dcm(2,2,:) = -sang(:,1).*cang(:,2).*sang(:,3) + cang(:,1).*cang(:,3);
        dcm(2,3,:) = cang(:,1).*cang(:,2).*sang(:,3) + sang(:,1).*cang(:,3);                
        dcm(3,1,:) = sang(:,2).*cang(:,3);        
        dcm(3,2,:) = -sang(:,1).*cang(:,3).*cang(:,2) - cang(:,1).*sang(:,3);
        dcm(3,3,:) = cang(:,1).*cang(:,3).*cang(:,2) - sang(:,1).*sang(:,3);
        
    case 'xzy'
        %     [          cy*cz, sz*cx*cy+sy*sx, cy*sx*sz-sy*cx]
        %     [            -sz,          cz*cx,          cz*sx]
        %     [          sy*cz, sy*cx*sz-cy*sx, sy*sx*sz+cy*cx]

        dcm(1,1,:) = cang(:,3).*cang(:,2);
        dcm(1,2,:) = cang(:,1).*cang(:,3).*sang(:,2) + sang(:,1).*sang(:,3);
        dcm(1,3,:) = sang(:,1).*cang(:,3).*sang(:,2) - cang(:,1).*sang(:,3);
        dcm(2,1,:) = -sang(:,2);
        dcm(2,2,:) = cang(:,1).*cang(:,2);
        dcm(2,3,:) = sang(:,1).*cang(:,2);        
        dcm(3,1,:) = sang(:,3).*cang(:,2);
        dcm(3,2,:) = cang(:,1).*sang(:,2).*sang(:,3) - sang(:,1).*cang(:,3);                
        dcm(3,3,:) = sang(:,1).*sang(:,2).*sang(:,3) + cang(:,1).*cang(:,3);
        
    case 'xzx'
        %     [                cz,             sz*cx,             sz*sx]
        %     [           -cx2*sz,  cx2*cz*cx-sx2*sx,  cx2*cz*sx+sx2*cx]
        %     [            sx2*sz, -sx2*cz*cx-cx2*sx, -sx2*cz*sx+cx2*cx]

        dcm(1,1,:) = cang(:,2);
        dcm(1,2,:) = cang(:,1).*sang(:,2);     
        dcm(1,3,:) = sang(:,1).*sang(:,2);
        dcm(2,1,:) = -sang(:,2).*cang(:,3);        
        dcm(2,2,:) = cang(:,1).*cang(:,3).*cang(:,2) - sang(:,1).*sang(:,3);
        dcm(2,3,:) = sang(:,1).*cang(:,3).*cang(:,2) + cang(:,1).*sang(:,3);
        dcm(3,1,:) = sang(:,2).*sang(:,3);
        dcm(3,2,:) = -cang(:,1).*cang(:,2).*sang(:,3) - sang(:,1).*cang(:,3);                
        dcm(3,3,:) = -sang(:,1).*cang(:,2).*sang(:,3) + cang(:,1).*cang(:,3);

    otherwise
        error(message('aero:angle2dcm:unknownRotation', type));
end

== matlab function GS_model/Subsystem2/Subsystem/Actuator/Magnetorquer/Mt_MathModel/MtA1/Saturation ==
  data: Mc_In input; Num input; Mc_Out output; Mt_max_M input
function Mc_Out = fcn(Mc_In,Num,Mt_max_M)
if Mc_In > Mt_max_M(Num)
    Mc_Out = Mt_max_M(Num);
elseif Mc_In < -Mt_max_M(Num)
    Mc_Out = -Mt_max_M(Num);
else
    Mc_Out = Mc_In;
end

== matlab function GS_model/Subsystem2/Subsystem/PhysicsModel/Environment/Air Torque Subsystem/Subsystem/MATLAB Function ==
  data: r input; lon output; lat output; h output
%--------------------------------------------------------------------------
%
% Geodetic: geodetic coordinates (Longitude [rad], latitude [rad],
%           altitude [m]) from given position vector (r [m])
%
% Last modified:   2018/01/27   M. Mahooti
% 
%--------------------------------------------------------------------------
function [lon, lat, h] = m_Geodetic(r)


R_equ = 6378136.3 ; 
f     = 0.00335281066474748;

epsRequ = 1e-9*R_equ;      % Convergence criterion
e2      = f*(2-f);        % Square of eccentricity

X = r(1);                 % Cartesian coordinates
Y = r(2);
Z = r(3);
rho2 = X*X + Y*Y;         % Square of distance from z-axis

% Check validity of input data
if (norm(r)==0)
    disp ( ' invalid input in Geodetic constructor\n' );
    lon = 0;
    lat = 0;
    h   = R_equ;
    return
end

% Iteration 
dZ = e2*Z;

while(1)
    ZdZ    = Z + dZ;
    Nh     = sqrt ( rho2 + ZdZ*ZdZ ); 
    SinPhi = ZdZ / Nh;    % Sine of geodetic latitude
    N      = R_equ / sqrt(1-e2*SinPhi*SinPhi);
    dZ_new = N*e2*SinPhi;
    if (abs(dZ-dZ_new) < epsRequ)
        break
    end
    dZ = dZ_new;
end

% Longitude, latitude, altitude
lon = atan2(Y, X);
lat = atan2(ZdZ, sqrt(rho2));
h   = Nh - N;

== matlab function GS_model/Subsystem2/Subsystem/PhysicsModel/Environment/Air Torque Subsystem/Subsystem/MATLAB Function1 ==
  data: height input; d_min output; d_max output; h input; c_min input; c_max input
%--------------------------------------------------------------------------
%
% Geodetic: geodetic coordinates (Longitude [rad], latitude [rad],
%           altitude [m]) from given position vector (r [m])
%
% Last modified:   2018/01/27   M. Mahooti
% 
%--------------------------------------------------------------------------
function [d_min,d_max] = m_para_cal(height,h,c_min,c_max)

height = height/1000;
% Height index search and exponential density interpolation
ih = 1;                           % section index reset
for  i=1:59-1                 % loop over N_Coef height regimes
  if ( height >= h(i) && height < h(i+1) )
    ih = i;                       % ih identifies height section
    break
  end
end
h_min = ( h(ih) - h(ih+1) )/log( c_min(ih+1)/c_min(ih) );
h_max = ( h(ih) - h(ih+1) )/log( c_max(ih+1)/c_max(ih) );

d_min = c_min(ih) * exp( (h(ih)-height)/h_min );
d_max = c_max(ih) * exp( (h(ih)-height)/h_max );

== matlab function GS_model/Subsystem2/Subsystem/PhysicsModel/Environment/MagneticCal/MATLAB Function ==
  data: LBH_Geocentric input; fRV input; Mag_VVLH output
% load data
% data=simout.data;
% RV=simout1.data;
% RV=reshape(RV,6,[])';
% [len,~]=size(data);
% Mag=zeros(len,8);
% 
% 
% 
% for i=1:len
%     Mag(i,:)=Mag_Cal(data(i,4:6), RV(i,:));
% end
function Mag_VVLH = Mag_Cal(LBH_Geocentric,fRV)
Long = LBH_Geocentric(1);% 算磁场用地心经纬度
theta=pi/2-LBH_Geocentric(2);


x=fRV(1);
y=fRV(2);
z=fRV(3);
vx=fRV(4);
vy=fRV(5);
vz=fRV(6);
r=norm([x,y,z]);
Z=[x,y,z];
Z=Z/r;
Y=cross([x,y,z],[vx,vy,vz]);
Y=Y/norm(Y);
X=cross(Y,Z);
A=[X;Y;Z];

EARTH_RADIUS_M=6371230;
re_r=EARTH_RADIUS_M/r;
re_r3=re_r*re_r*re_r;
re_r4=re_r3*re_r;
re_r5=re_r4*re_r;
sin_theta=sin(theta);
cos_theta=cos(theta);
sin_2theta=sin(2.0*theta);
cos_2theta=cos(2.0*theta);
sin_lambdal=sin(Long);
cos_lambdal=cos(Long);
sin_2lambdal=sin(2.0*Long);
sin_3lambdal=sin(3.0*Long);
cos_2lambdal=cos(2.0*Long);
cos_3lambdal=cos(3.0*Long);
sin2_theta=sin_theta*sin_theta;
sin3_theta=sin2_theta*sin_theta;
cos2_theta=cos_theta*cos_theta;
cos3_theta=cos2_theta*cos_theta;
G10=-29404.8;G11=-1450.9;H11=4652.5;
G20=-2499.6;G21=2982.0;H21=-2991.6;G22=1677.0;H22=-734.6;
G30=1363.2;G31=-2381.2;H31=-82.1;G32=1236.2;H32=241.9;
G33=525.7;H33=-543.4;
SQRT3=sqrt(3);
HALFSQRT3=sqrt(3)/2;
SQRT6D4=sqrt(6)/4;
HALFSQRT15=sqrt(15)/2;
SQRT10M3D4=sqrt(10)*3/4;
SQRT10D4=sqrt(10)/4;
re3_f64=(G10*(-sin_theta)+(G11*cos_lambdal+H11*sin_lambdal)*cos_theta);
re4_f64=(G20*(-3.0*sin_theta*cos_theta)+...
(G21*cos_lambdal+H21*sin_lambdal)*(SQRT3*cos_2theta)+...
(G22*cos_2lambdal+H22*sin_2lambdal)*(HALFSQRT3*sin_2theta));
re5_f64=(G30*(1.5*sin_theta*(1.0-5.0*cos2_theta))+...
(G31*cos_lambdal+H31*sin_lambdal)*(SQRT6D4*cos_theta*(4.0-15.0*sin2_theta))+...
(G32*cos_2lambdal+H32*sin_2lambdal)*(HALFSQRT15*sin_theta*(3.0*cos2_theta-1.0))+...
(G33*cos_3lambdal+H33*sin_3lambdal)*(SQRT10M3D4*sin2_theta*cos_theta));
bn=re_r3*re3_f64+re_r4*re4_f64+re_r5*re5_f64;
re3_f64=((G11*sin_lambdal-H11*cos_lambdal)*sin_theta);
re4_f64=((G21*sin_lambdal-H21*cos_lambdal)*(HALFSQRT3*sin_2theta)+...
2.0*(G22*sin_2lambdal-H22*cos_2lambdal)*(HALFSQRT3*sin2_theta));
re5_f64=((G31*sin_lambdal-H31*cos_lambdal)*(SQRT6D4*sin_theta*(5.0*cos2_theta-1.0))+...
2.0*(G32*sin_2lambdal-H32*cos_2lambdal)*(HALFSQRT15*sin2_theta*cos_theta)+...
3.0*(G33*sin_3lambdal-H33*cos_3lambdal)*(SQRT10D4*sin3_theta));

Mag_VVLH = [0;0;0];
if sin_theta~=0.0
    be=1.0/sin_theta*(re_r3*re3_f64+re_r4*re4_f64+re_r5*re5_f64);
    re3_f64=(G10*cos_theta+(G11*cos_lambdal+H11*sin_lambdal)*sin_theta);
    re4_f64=(G20*(1.5*cos2_theta-0.5)+...
    (G21*cos_lambdal+H21*sin_lambdal)*(HALFSQRT3*sin_2theta)+...
    (G22*cos_2lambdal+H22*sin_2lambdal)*(HALFSQRT3*sin2_theta));
    re5_f64=(G30*(2.5*cos3_theta-1.5*cos_theta)+...
    (G31*cos_lambdal+H31*sin_lambdal)*(SQRT6D4*sin_theta*(5.0*cos2_theta-1.0))+...
    (G32*cos_2lambdal+H32*sin_2lambdal)*(HALFSQRT15*sin2_theta*cos_theta)+...
    (G33*cos_3lambdal+H33*sin_3lambdal)*(SQRT10D4*sin3_theta));
    bg=-2.0*re_r3*re3_f64-3.0*re_r4*re4_f64-4.0*re_r5*re5_f64;
    
    
    vn=(-z*(x*vx+y*vy)+(x*x+y*y)*vz)/r/sqrt(x*x+y*y);
    ve=(-y*vx+x*vy)/sqrt(x*x+y*y);
    vh=norm([vn,ve]);
    vn=vn/vh;
    ve=ve/vh;
    aon_m33=[vn ve 0;-ve vn 0;0 0 1];
    Mag_NEG=[bn;be;bg]*1.0e-5; % Gs
    Mag_VVLH=aon_m33*Mag_NEG;
end
end

== matlab function GS_model/Subsystem2/Subsystem/Actuator/Magnetorquer/Mt_MathModel/MtA2/Saturation ==
  data: Mc_In input; Num input; Mc_Out output; Mt_max_M input
function Mc_Out = fcn(Mc_In,Num,Mt_max_M)
if Mc_In > Mt_max_M(Num)
    Mc_Out = Mt_max_M(Num);
elseif Mc_In < -Mt_max_M(Num)
    Mc_Out = -Mt_max_M(Num);
else
    Mc_Out = Mc_In;
end

== matlab function GS_model/Subsystem2/Subsystem/Actuator/Magnetorquer/Mt_MathModel/MtA3/Saturation ==
  data: Mc_In input; Num input; Mc_Out output; Mt_max_M input
function Mc_Out = fcn(Mc_In,Num,Mt_max_M)
if Mc_In > Mt_max_M(Num)
    Mc_Out = Mt_max_M(Num);
elseif Mc_In < -Mt_max_M(Num)
    Mc_Out = -Mt_max_M(Num);
else
    Mc_Out = Mc_In;
end

== matlab function GS_model/Subsystem2/ /Subsystem/MATLAB Function ==
  data: AssA input; Ass_Tm output; AssB input; AssC input; AssD input; AssE input; AssF input; Ass_TmOrder input
function Ass_Tm = fcn(AssA,AssB,AssC,AssD,AssE,AssF,Ass_TmOrder)
Ass = [AssA AssB AssC AssD AssE AssF];
Ass_Tm = zeros(24,1);
for i = 1:6
    Ass_Tm((i-1)*4+1:i*4,1) = Ass(:,Ass_TmOrder(i));
end

== matlab function GS_model/Subsystem2/Subsystem/Actuator/Magnetorquer/Mt_MathModel/MtA4/Saturation ==
  data: Mc_In input; Num input; Mc_Out output; Mt_max_M input
function Mc_Out = fcn(Mc_In,Num,Mt_max_M)
if Mc_In > Mt_max_M(Num)
    Mc_Out = Mt_max_M(Num);
elseif Mc_In < -Mt_max_M(Num)
    Mc_Out = -Mt_max_M(Num);
else
    Mc_Out = Mc_In;
end

== matlab function GS_model/Subsystem2/Subsystem/PhysicsModel/Subsystem3/Subsystem1/MATLAB Function ==
  data: Agl input; A output; Order input
function A = Agl2DCM(Agl,Order)
% 输入：(1)转序，123或213等
%      (2)转角，按照转序顺序排列，如213转序角度顺序为[YXZ];
A = eye(3);
Num = size(Agl,1);
for i = 1:Num
    if Order(i) == 1
        A1 = Rx(Agl(i));
    elseif Order(i) == 2
        A1 = Ry(Agl(i));
    else
        A1 = Rz(Agl(i));
    end
    A = A1*A;
end
end
function A = Rx(alpha)
A = [1 0 0;0 cos(alpha) sin(alpha);0 -sin(alpha) cos(alpha)];
end
function A = Ry(alpha)
A = [cos(alpha) 0 -sin(alpha);0 1 0;sin(alpha) 0 cos(alpha)];
end
function A = Rz(alpha)
A = [cos(alpha) sin(alpha) 0;-sin(alpha) cos(alpha) 0;0 0 1];
end

== matlab function GS_model/Subsystem2/Subsystem/Actuator/Magnetorquer/Mt_MathModel/MtA5/Saturation ==
  data: Mc_In input; Num input; Mc_Out output; Mt_max_M input
function Mc_Out = fcn(Mc_In,Num,Mt_max_M)
if Mc_In > Mt_max_M(Num)
    Mc_Out = Mt_max_M(Num);
elseif Mc_In < -Mt_max_M(Num)
    Mc_Out = -Mt_max_M(Num);
else
    Mc_Out = Mc_In;
end

== matlab function GS_model/Subsystem2/Subsystem/Actuator/Magnetorquer/Mt_MathModel/MtA6/Saturation ==
  data: Mc_In input; Num input; Mc_Out output; Mt_max_M input
function Mc_Out = fcn(Mc_In,Num,Mt_max_M)
if Mc_In > Mt_max_M(Num)
    Mc_Out = Mt_max_M(Num);
elseif Mc_In < -Mt_max_M(Num)
    Mc_Out = -Mt_max_M(Num);
else
    Mc_Out = Mc_In;
end

== matlab function GS_model/Subsystem2/Subsystem/PhysicsModel/Subsystem3/Subsystem1/MATLAB Function1 ==
  data: Agl input; A output; Order input
function A = Agl2DCM(Agl,Order)
% 输入：(1)转序，123或213等
%      (2)转角，按照转序顺序排列，如312转序角度顺序为[zxy];
A = eye(3);
Num = size(Agl,1);
for i = 1:Num
    if Order(i) == 1
        A1 = Rx(Agl(i));
    elseif Order(i) == 2
        A1 = Ry(Agl(i));
    else
        A1 = Rz(Agl(i));
    end
    A = A1*A;
end
end
function A = Rx(alpha)
A = [1 0 0;0 cos(alpha) sin(alpha);0 -sin(alpha) cos(alpha)];
end
function A = Ry(alpha)
A = [cos(alpha) 0 -sin(alpha);0 1 0;sin(alpha) 0 cos(alpha)];
end
function A = Rz(alpha)
A = [cos(alpha) sin(alpha) 0;-sin(alpha) cos(alpha) 0;0 0 1];
end
